simulink library "wt_blockset_beta"  (Simulink 5.0)
values from neighbouring files (symbols this model uses):
  a = -Le\Re    [matrix_coeff_trafo3limb_abc.m]
  a11 = K2*Rs/Ls    [matrix_coeff_scim_abc.m]    (also in matrix_coeff_spsm_dq.m = -Rs*Ksgm_frd/Ksgm_d; matrix_coeff_trafo_abc.m = K2*Rhv/Lhv; matrix_coeff_wrim_abc.m)
  a12 = K3*Rs/Ls    [matrix_coeff_scim_abc.m]    (also in matrix_coeff_spsm_dq.m = Lssq*Ksgm_frd/Ksgm_d; matrix_coeff_trafo_abc.m = K3*Rhv/Lhv; matrix_coeff_wrim_abc.m)
  a13 = 3*Msr*sqrt(3)*K4/4    [matrix_coeff_scim_abc.m]    (also in matrix_coeff_spsm_dq.m = Rf*Lsgm_rd*Lmd/Ksgm_d; matrix_coeff_trafo_abc.m = K4*Rhv; matrix_coeff_wrim_abc.m)
  a14 = K4*Rr    [matrix_coeff_scim_abc.m]    (also in matrix_coeff_spsm_dq.m = Rrd*Lsgm_f*Lmd/Ksgm_d; matrix_coeff_trafo_abc.m = K2/Lhv; matrix_coeff_wrim_abc.m)
  a15 = Msr*(K2-K3)/Ls    [matrix_coeff_scim_abc.m]    (also in matrix_coeff_spsm_dq.m = Lmq*Ksgm_frd/Ksgm_d; matrix_coeff_trafo_abc.m = K3/Lhv; matrix_coeff_wrim_abc.m)
  a16 = K2/Ls    [matrix_coeff_scim_abc.m]    (also in matrix_coeff_spsm_dq.m = Ksgm_frd/Ksgm_d; matrix_coeff_trafo_abc.m = K4; matrix_coeff_wrim_abc.m)
  a17 = K3/Ls    [matrix_coeff_scim_abc.m]    (also in matrix_coeff_spsm_dq.m = -Lsgm_rd*Lmd/Ksgm_d; matrix_coeff_wrim_abc.m)
  a21 = -Lssd*Lsrq/Ksgm_q    [matrix_coeff_spsm_dq.m]
  a22 = -Rs*Lsrq/Ksgm_q    [matrix_coeff_spsm_dq.m]
  a23 = -Lsrq*Lmd/Ksgm_q    [matrix_coeff_spsm_dq.m]
  a24 = -Lsrq*Lmd/Ksgm_q    [matrix_coeff_spsm_dq.m]
  a25 = Rrq*Lmq/Ksgm_q    [matrix_coeff_spsm_dq.m]
  a26 = Lsrq/Ksgm_q    [matrix_coeff_spsm_dq.m]
  a31 = K4*Rs    [matrix_coeff_scim_abc.m]    (also in matrix_coeff_spsm_dq.m = +Rs*Lsgm_rd*Lmd/Ksgm_d; matrix_coeff_trafo_abc.m = K4*Rlv; matrix_coeff_wrim_abc.m)
  a32 = Msr*(K2-K3)/Lr    [matrix_coeff_scim_abc.m]    (also in matrix_coeff_spsm_dq.m = -Lssq*Lsgm_rd*Lmd/Ksgm_d; matrix_coeff_trafo_abc.m = K2*Rlv/Llv; matrix_coeff_wrim_abc.m)
  a33 = K2*Rr/Lr    [matrix_coeff_scim_abc.m]    (also in matrix_coeff_spsm_dq.m = -Rf*Ksgm_srd/Ksgm_d; matrix_coeff_trafo_abc.m = K3*Rlv/Llv; matrix_coeff_wrim_abc.m)
  a34 = K3*Rr/Lr    [matrix_coeff_scim_abc.m]    (also in matrix_coeff_spsm_dq.m = Rrd*Lsgm_s*Lmd/Ksgm_d; matrix_coeff_trafo_abc.m = K4; matrix_coeff_wrim_abc.m)
  a35 = 3*Msr*sqrt(3)*K4/4    [matrix_coeff_scim_abc.m]    (also in matrix_coeff_spsm_dq.m = -Lsgm_rd*Lmd*Lmq/Ksgm_d; matrix_coeff_trafo_abc.m = K2/Llv; matrix_coeff_wrim_abc.m)
  a36 = K4    [matrix_coeff_scim_abc.m]    (also in matrix_coeff_spsm_dq.m = -Lsgm_rd*Lmd/Ksgm_d; matrix_coeff_trafo_abc.m = K3/Llv; matrix_coeff_wrim_abc.m)
  a37 = Ksgm_srd/Ksgm_d    [matrix_coeff_spsm_dq.m]    (also in matrix_coeff_wrim_abc.m = K2/Lr)
  a41 = Rs*Lsgm_f*Lmd/Ksgm_d    [matrix_coeff_spsm_dq.m]
  a42 = -Lsgm_f*Lssq*Lmd/Ksgm_d    [matrix_coeff_spsm_dq.m]
  a43 = Rf*Lsgm_s*Lmd/Ksgm_d    [matrix_coeff_spsm_dq.m]
  a44 = -Rrd*Ksgm_sf/Ksgm_d    [matrix_coeff_spsm_dq.m]
  a45 = -Lsgm_f*Lmd*Lmq/Ksgm_d    [matrix_coeff_spsm_dq.m]
  a46 = -Lsgm_f*Lmd/Ksgm_d    [matrix_coeff_spsm_dq.m]
  a47 = -Lsgm_s*Lmd/Ksgm_d    [matrix_coeff_spsm_dq.m]
  a51 = Lssd*Lmq/Ksgm_q    [matrix_coeff_spsm_dq.m]
  a52 = Rs*Lmq/Ksgm_q    [matrix_coeff_spsm_dq.m]
  a53 = Lmd*Lmq/Ksgm_q    [matrix_coeff_spsm_dq.m]
  a54 = Lmd*Lmq/Ksgm_q    [matrix_coeff_spsm_dq.m]
  a55 = -Rrq*Lssq/Ksgm_q    [matrix_coeff_spsm_dq.m]
  a56 = -Lmq/Ksgm_q    [matrix_coeff_spsm_dq.m]
  alpha_T = Ubase_hv/Ubase_lv    [matrix_coeff_trafo3limb_abc.m]
  b = inv(Le)    [matrix_coeff_trafo3limb_abc.m]
  Ctorque = cq(2:5:102,2:5:182)    [cq_table.m]
  Lmd = mag_ind(1)    [matrix_coeff_spsm_dq.m]
  Lmq = mag_ind(2)    [matrix_coeff_spsm_dq.m]
  Lss = Lsgms+Lm    [init_dbe_dq_scim.m]
  omg_base = 2*pi*rated_fp(1)    [init_dbe_dq_scim.m]    (also in init_dbe_rms_scim.m)
  p = rated_fp(2)    [init_dbe_dq_scim.m]    (also in init_dbe_rms_scim.m)
  Rs = stator(1)    [init_dbe_dq_scim.m]    (also in init_dbe_rms_scim.m; matrix_coeff_scim_abc.m; matrix_coeff_spsm_dq.m = stator_winding(1); matrix_coeff_wrim_abc.m)
  Xs = omg_base*Lss    [init_dbe_dq_scim.m]    (also in init_dbe_rms_scim.m = Xsgm_s+Xm)
undefined symbols (not defined in the file or in its folder): get, j, Kmode, ModeOp, Type, u0
libraries: simulink_extras x12, simulink x4, dspinverses x1, dspmtrx3 x1, dspsigattribs x1, dspspect3 x1
(part 2 of 4)

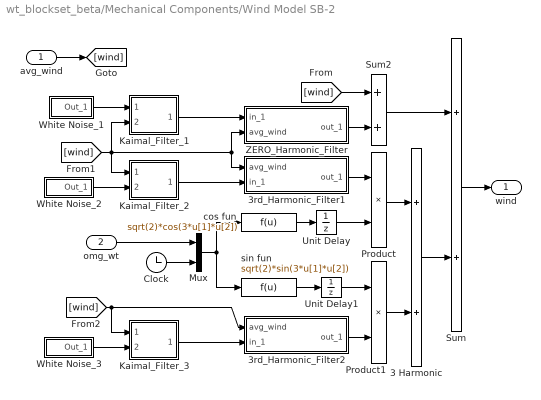
== system wt_blockset_beta/Mechanical Components/Wind Model SB-2 ==
  avg_wind : Inport
  omg_wt : Inport  Port=2
  3 Harmonic : Sum  SaturateOnIntegerOverflow=on  InputSameDT=on
  3rd_Harmonic_Filter1 : Subsystem
  3rd_Harmonic_Filter2 : Subsystem
  Clock : Clock
  Kaimal_Filter_1 : Subsystem
  Kaimal_Filter_2 : Subsystem
  Kaimal_Filter_3 : Subsystem
  Mux : Mux  Inputs=2
  Product : Product  SaturateOnIntegerOverflow=on  InputSameDT=on
  Product1 : Product  SaturateOnIntegerOverflow=on  InputSameDT=on
  Sum : Sum  SaturateOnIntegerOverflow=on  InputSameDT=on
  Sum2 : Sum  SaturateOnIntegerOverflow=on  InputSameDT=on
  Unit Delay : UnitDelay  SampleTime=T_sample
  Unit Delay1 : UnitDelay  SampleTime=T_sample
  White Noise_1 : Subsystem  mask(Continuous White Noise.){Cov=[1], Ts=T_sample, seed=[256]}
      mask prompts: Cov "Noise Power:"; Ts "Sample Time:"
      mask help:
      | White noise for continuous (s-domain) systems.
      | Band-limited using zero-order-hold.
      mask init:
      | r = rand(1,12); r2 = [r(1),r;r,r(12)]; t =[1:13;1:13];
      mask Help: Implemented using white noise into Zero-Order Hold block. The seed and power can be vectors of the same length to produce a vector of white noise sources. For faster simulation, set sample time to the highest value possible but in accordance with the fastest dynamics of system.
      mask Display: plot(t(:),r2(:))
  White Noise_2 : Subsystem  mask(Continuous White Noise.){@1=[1], @2=T_sample, @3=[894]}
      mask prompts: @1 "Noise Power:"; @2 "Sample Time:"; @3 "Seed"
      mask help:
      | White noise for continuous (s-domain) systems.
      | Band-limited using zero-order-hold.
      mask init:
      | Cov = @1; Ts = @2; seed = @3; r = rand(1,12); r2 = [r(1),r;r,r(12)]; t =[1:13;1:13];
      mask Help: Implemented using white noise into Zero-Order Hold block. The seed and power can be vectors of the same length to produce a vector of white noise sources. For faster simulation, set sample time to the highest value possible but in accordance with the fastest dynamics of system.
      mask Display: plot(t(:),r2(:))
  White Noise_3 : Subsystem  mask(Continuous White Noise.){@1=[1], @2=T_sample, @3=[31]}
      mask prompts: @1 "Noise Power:"; @2 "Sample Time:"; @3 "Seed"
      mask help:
      | White noise for continuous (s-domain) systems.
      | Band-limited using zero-order-hold.
      mask init:
      | Cov = @1; Ts = @2; seed = @3; r = rand(1,12); r2 = [r(1),r;r,r(12)]; t =[1:13;1:13];
      mask Help: Implemented using white noise into Zero-Order Hold block. The seed and power can be vectors of the same length to produce a vector of white noise sources. For faster simulation, set sample time to the highest value possible but in accordance with the fastest dynamics of system.
      mask Display: plot(t(:),r2(:))
  ZERO_Harmonic_Filter : Subsystem
  cos fun : Fcn  Expr=sqrt(2)*cos(3*u[1]*u[2])
  sin fun : Fcn  Expr=sqrt(2)*sin(3*u[1]*u[2])
  wind : Outport  InitialOutput=[u0]
  wires:
  Clock/1 -> Mux/2
  Unit Delay1/1 -> Product1/1
  Unit Delay/1 -> Product/2
  omg_wt/1 -> Mux/1
  Mux/1 -> sin fun/1, cos fun/1
  3rd_Harmonic_Filter1/1(out_1) -> Product/1
  White Noise_3/1(Out_1) -> Kaimal_Filter_3/2(in_1)
  White Noise_1/1(Out_1) -> Kaimal_Filter_1/1(in_1)
  Sum/1 -> wind/1
  [wind] -> Sum2/1
  Sum2/1 -> Sum/1
  ZERO_Harmonic_Filter/1(out_1) -> Sum2/2
  3 Harmonic/1 -> Sum/2
  3rd_Harmonic_Filter2/1(out_1) -> Product1/2
  Product1/1 -> 3 Harmonic/2
  Product/1 -> 3 Harmonic/1
  sin fun/1 -> Unit Delay1/1
  cos fun/1 -> Unit Delay/1
  Kaimal_Filter_1/1(out_1) -> ZERO_Harmonic_Filter/1(in_1)
  Kaimal_Filter_2/1(out_1) -> 3rd_Harmonic_Filter1/2(in_1)
  White Noise_2/1(Out_1) -> Kaimal_Filter_2/2(in_1)
  avg_wind/1 -> [wind]
  [wind] -> Kaimal_Filter_1/2(avg_wind), Kaimal_Filter_2/1(avg_wind), ZERO_Harmonic_Filter/2(avg_wind), 3rd_Harmonic_Filter1/1(avg_wind)
  [wind] -> Kaimal_Filter_3/1(avg_wind), 3rd_Harmonic_Filter2/1(avg_wind)
  Kaimal_Filter_3/1(out_1) -> 3rd_Harmonic_Filter2/2(in_1)

== system wt_blockset_beta/Mechanical Components/Wind Turbine Rotor ==
  pitch : Inport
  wind : Inport  Port=2
  omg_wt : Inport  Port=3
  Actuator : TransferFcn  Denominator=[Tact 1]
  Logical Operator : Logic
  Look-Up Table (n-D) : S-Function  FunctionName=sfun_lookupnd  Parameters=numDims,tableData,bp1,bp2,bp3,bp4,bpcell,searchMode,cacheBpFlag,vectorInputFlag,interpMethod,extrapMethod,rangeErrorMode  mask(LookupNDInterp){numDimsPopupSelect=2, bp1=[0:1:20], bp2=[-90:5:90], bp3=[1:3], bp4=[1:3], bpcell={ [1:3], [1:3] }, explicitNumDims=2, searchMode=Binary Search, cacheBpFlag=off, vectorInputFlag=off, tableData=Ctorque, interpMethod=Linear, extrapMethod=None - Clip, rangeErrorMode=Error}
      mask prompts: numDimsPopupSelect "Number of table dimensions:"; bp1 "First input (row) breakpoint set:"; bp2 "Second (column) input breakpoint set:"; bp3 "Third input breakpoint set:"; bp4 "Fourth input breakpoint set:"; bpcell "Fifth..Nth breakpoint sets (cell array):"; explicitNumDims "Explicit number of dimensions:"; searchMode "Index search method:"; cacheBpFlag "Begin index searches using previous index results"; vectorInputFlag "Use one (vector) input port instead of N ports"; tableData "Table data:"; interpMethod "Interpolation method:"; extrapMethod "Extrapolation method:"; rangeErrorMode "Action for out of range input:"
      mask help: Perform n-dimensional interpolated table lookup including index searches. The table is a sampled representation of a function in N variables. Breakpoint sets relate the input values to positions in the table. The first dimension corresponds to the top (or left) input port.
      mask init:
      | if numDimsPopupSelect==5
      |   numDims=explicitNumDims;
      | else
      |   numDims=numDimsPopupSelect;
      | end
      | if strcmp(get_param(bdroot(gcb),'BlockDiagramType'),'library')
      |   dimsChar = 'n';
      | else
      |   dimsChar = sprintf('%d',numDims);
      | end
      | switch interpMethod
      |   case 1
      |     plottype = 'flatplot';
      |   case 2
      |     plottype = 'lineplot';
      |   otherwise
      |     plottype = 'splineplot';
      | end
      | for i=1:numDims
      |   switch( i )
      |     case 1
      |       bp = bp1;
      |     case 2
      |       bp = bp2;
      |     case 3
      |       bp = bp3;
      |     case 4
      |       bp = bp4;
      |     otherwise
      |       bp = bpcell{i-4};
      |    end
      |    Lbp = length(bp);
      |    if i < 2
      |      bpData = reshape(bp,Lbp,1);
      |      bpIndices = 0;
      |    else
      |      bpData = [ bpData; reshape(bp,Lbp,1) ];
      |      bpIndices = [ bpIndices; bpIndices(i-1)+LbpPrev ];
      |    end
      |    LbpPrev = Lbp;
      | end
      | [x,y,xaxes,yaxes] = ndlookico(plottype, numDims,{bpData,bpIndices,tableData});
      mask StyleString: popup(   1   |   2   |   3   |   4   |More...),edit,edit,edit,edit,edit,edit,popup(Evenly Spaced Points|Linear Search|Binary Search),checkbox,checkbox,edit,popup(None - Flat|Linear|Cubic Spline),popup(None - Clip|Linear|Cubic Spline),popup(None|Warning|Error)
      mask CallbackString: ndlookico|||||||||||||
      mask Display:
      | text(0.5,0.9,sprintf(' %s-D T(u)',dimsChar),'horizontalAlignment','center')
      | plot(x,y)
      | plot(xaxes,yaxes)
  Mux : Mux  Inputs=2
  Mux1 : Mux  Inputs=2
  Relational Operator : RelationalOperator  InputSameDT=on
  Relational Operator1 : RelationalOperator  Operator=<=  InputSameDT=on
  Switch : Switch  Threshold=.5  SaturateOnIntegerOverflow=on  InputSameDT=on
  Torque : Fcn  Expr=-0.5*pi*ro_air*(R^3)*(u(1)^2)*u(2)
  cut_in : Constant  Value=cut_in
  cut_out : Constant  Value=cut_out
  lamda : Fcn  Expr=u(2)*R/u(1)
  null : Constant  Value=0
  T_wt : Outport
  wires:
  pitch/1 -> Actuator/1
  lamda/1 -> Look-Up Table (n-D)/1
  Look-Up Table (n-D)/1 -> Mux1/2
  wind/1 -> Mux1/1, Relational Operator1/1, Relational Operator/1, Mux/1
  Logical Operator/1 -> Switch/2
  null/1 -> Switch/3
  Torque/1 -> Switch/1
  Switch/1 -> T_wt/1
  Relational Operator/1 -> Logical Operator/1
  Relational Operator1/1 -> Logical Operator/2
  cut_out/1 -> Relational Operator1/2
  cut_in/1 -> Relational Operator/2
  omg_wt/1 -> Mux/2
  Mux1/1 -> Torque/1
  Mux/1 -> lamda/1
  Actuator/1 -> Look-Up Table (n-D)/2

== system wt_blockset_beta/Power Converters/3-phase Diode Bridge Rectifier ==
  note: Phase Voltage
  note: Phase Current
  note: DC-link Current
  v_ph : Inport
  Idc : Inport  Port=2
  DC-link Voltage : Fcn  Expr=u(1)+u(2)+u(3)
  Diode  State Calculator : Subsystem
  Product1 : Product  SaturateOnIntegerOverflow=on  InputSameDT=on
  Product3 : Product  SaturateOnIntegerOverflow=on  InputSameDT=on
  i_ph : Outport  InitialOutput=0
  Vdc : Outport  Port=2  InitialOutput=0
  wires:
  v_ph/1 -> Diode  State Calculator/1(RST), Product3/1
  Product3/1 -> DC-link Voltage/1
  DC-link Voltage/1 -> Vdc/1
  Diode  State Calculator/1(K) -> Product3/2, Product1/1
  Idc/1 -> Product1/2
  Product1/1 -> i_ph/1

== system wt_blockset_beta/Power Converters/Average PWM Strategy ==
  vd_ref : Inport
  vq_ref : Inport  Port=2
  Vdc : Inport  Port=3
  freq : Inport  Port=4
  Gain : Gain  Gain=2*pi  SaturateOnIntegerOverflow=on
  Integrator : Integrator
  Mux : Mux  Inputs=2
  Mux1 : Mux  Inputs=3
  Mux2 : Mux  Inputs=3
  duty_A1 : Fcn  Expr=0.5*2/sqrt(3)*u(1)*(sin(u(2))+(sin(3*u(2))/6)*(third==1))
  duty_A2 : Fcn  Expr=0.5*2/sqrt(3)*u(1)*(sin(u(2)-2*pi/3)+(sin(3*u(2))/6)*(third==1))
  duty_A3 : Fcn  Expr=0.5*2/sqrt(3)*u(1)*(sin(u(2)+2*pi/3)+(sin(3*u(2))/6)*(third==1))
  ma : Fcn  Expr=sqrt(3)/2*sqrt(u(1)^2+u(3)^2)/u(2)
  duty_ABC : Outport
  wires:
  freq/1 -> Gain/1
  Mux/1 -> duty_A1/1, duty_A2/1, duty_A3/1
  Integrator/1 -> Mux/2
  Gain/1 -> Integrator/1
  duty_A1/1 -> Mux1/1
  duty_A2/1 -> Mux1/2
  duty_A3/1 -> Mux1/3
  Mux2/1 -> ma/1
  ma/1 -> Mux/1
  vd_ref/1 -> Mux2/1  "vdref"
  Vdc/1 -> Mux2/2  "vdc"
  vq_ref/1 -> Mux2/3  "vqref"
  Mux1/1 -> duty_ABC/1

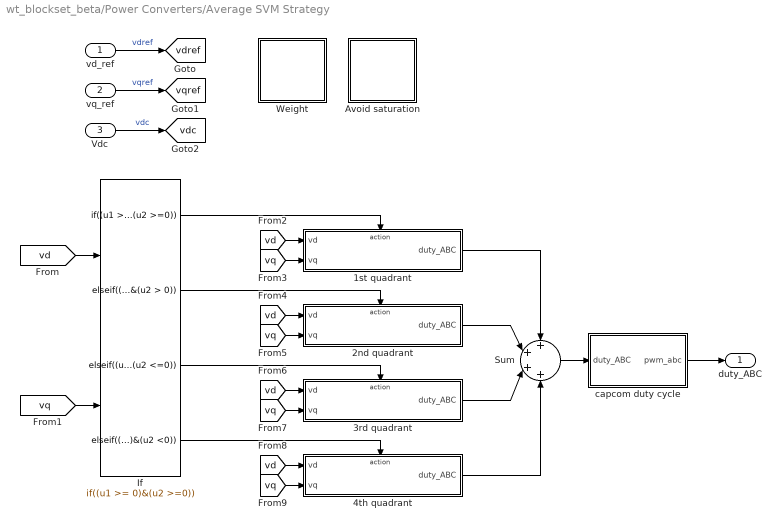
== system wt_blockset_beta/Power Converters/Average SVM Strategy ==
  vd_ref : Inport
  vq_ref : Inport  Port=2
  Vdc : Inport  Port=3
  1st quadrant : Subsystem  TreatAsAtomicUnit=on
  2nd quadrant : Subsystem  TreatAsAtomicUnit=on
  3rd quadrant : Subsystem  TreatAsAtomicUnit=on
  4th quadrant : Subsystem  TreatAsAtomicUnit=on
  "Avoid saturation " : Subsystem
      mask Display: disp('Avoid\nSaturation')
  If : If  NumInputs=2  IfExpression=(u1 >= 0)&(u2 >=0)  ElseIfExpressions=(u1 < 0)&(u2 > 0), (u1 < 0)&(u2 <=0), (u1 >= 0)&(u2 <0)  ShowElse=off
  Sum : Sum  Inputs=++++  SaturateOnIntegerOverflow=on
  Weight : Subsystem
      mask Type: Avoid saturation
      mask Display: disp('Weight')
  capcom duty cycle : Subsystem
  duty_ABC : Outport
  tag scope: vdc=global, vdref=global, vqref=global
  wires:
  vd_ref/1 -> [vdref]  "vdref"
  vq_ref/1 -> [vqref]  "vqref"
  Vdc/1 -> [vdc]  "vdc"
  [vd] -> If/1
  [vq] -> If/2
  If/1 -> 1st quadrant/Action
  [vd] -> 1st quadrant/1(vd)
  [vq] -> 1st quadrant/2(vq)
  [vd] -> 2nd quadrant/1(vd)
  [vq] -> 2nd quadrant/2(vq)
  If/2 -> 2nd quadrant/Action
  [vd] -> 3rd quadrant/1(vd)
  [vq] -> 3rd quadrant/2(vq)
  If/3 -> 3rd quadrant/Action
  [vd] -> 4th quadrant/1(vd)
  [vq] -> 4th quadrant/2(vq)
  If/4 -> 4th quadrant/Action
  1st quadrant/1(duty_ABC) -> Sum/1
  2nd quadrant/1(duty_ABC) -> Sum/2
  4th quadrant/1(duty_ABC) -> Sum/4
  3rd quadrant/1(duty_ABC) -> Sum/3
  Sum/1 -> capcom duty cycle/1(duty_ABC)
  capcom duty cycle/1(pwm_abc) -> duty_ABC/1

== system wt_blockset_beta/Power Converters/Switching PWM Strategy ==
  vd_ref : Inport
  vq_ref : Inport  Port=2
  Vdc : Inport  Port=3
  freq : Inport  Port=4
  Gain : Gain  Gain=2*pi  SaturateOnIntegerOverflow=on
  Integrator : Integrator
  Mux : Mux  Inputs=2
  Mux1 : Mux  Inputs=3
  Mux2 : Mux  Inputs=3
  capcom : Subsystem
  dead_time_A : Subsystem
  duty_A1 : Fcn  Expr=0.5*2/sqrt(3)*u(1)*(sin(u(2))+(sin(3*u(2))/6)*(third==1))
  duty_A2 : Fcn  Expr=0.5*2/sqrt(3)*u(1)*(sin(u(2)-2*pi/3)+(sin(3*u(2))/6)*(third==1))
  duty_A3 : Fcn  Expr=0.5*2/sqrt(3)*u(1)*(sin(u(2)+2*pi/3)+(sin(3*u(2))/6)*(third==1))
  ma : Fcn  Expr=sqrt(3)/2*sqrt(u(1)^2+u(3)^2)/u(2)
  pulse dropping : Subsystem
  Sw_ABC : Outport
  wires:
  vq_ref/1 -> Mux2/3  "vqref"
  Vdc/1 -> Mux2/2  "vdc"
  vd_ref/1 -> Mux2/1  "vdref"
  ma/1 -> Mux/1
  Mux2/1 -> ma/1
  duty_A3/1 -> Mux1/3
  duty_A2/1 -> Mux1/2
  duty_A1/1 -> Mux1/1
  Gain/1 -> Integrator/1
  Integrator/1 -> Mux/2
  Mux/1 -> duty_A3/1, duty_A2/1, duty_A1/1
  freq/1 -> Gain/1
  capcom/1(S_ABC) -> dead_time_A/1(pwm_A)
  Mux1/1 -> pulse dropping/1(duty_ABC)
  pulse dropping/1(duty_abc) -> capcom/1(duty_abc)
  dead_time_A/1(S_A) -> Sw_ABC/1

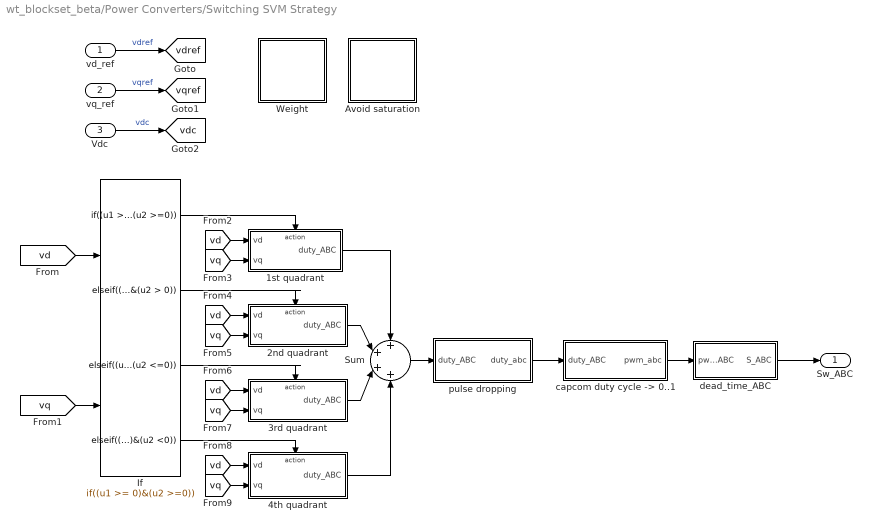
== system wt_blockset_beta/Power Converters/Switching SVM Strategy ==
  vd_ref : Inport
  vq_ref : Inport  Port=2
  Vdc : Inport  Port=3
  1st quadrant : Subsystem  TreatAsAtomicUnit=on
  2nd quadrant : Subsystem  TreatAsAtomicUnit=on
  3rd quadrant : Subsystem  TreatAsAtomicUnit=on
  4th quadrant : Subsystem  TreatAsAtomicUnit=on
  "Avoid saturation " : Subsystem
      mask Display: disp('Avoid\nSaturation')
  If : If  NumInputs=2  IfExpression=(u1 >= 0)&(u2 >=0)  ElseIfExpressions=(u1 < 0)&(u2 > 0), (u1 < 0)&(u2 <=0), (u1 >= 0)&(u2 <0)  ShowElse=off
  Sum : Sum  Inputs=++++  SaturateOnIntegerOverflow=on
  Weight : Subsystem
      mask Type: Avoid saturation
      mask Display: disp('Weight')
  "capcom duty cycle -> 0..1" : Subsystem
  dead_time_ABC : Subsystem
  pulse dropping : Subsystem
  Sw_ABC : Outport
  tag scope: vdc=global, vdref=global, vqref=global
  wires:
  vd_ref/1 -> [vdref]  "vdref"
  vq_ref/1 -> [vqref]  "vqref"
  Vdc/1 -> [vdc]  "vdc"
  [vd] -> If/1
  [vq] -> If/2
  If/1 -> 1st quadrant/Action
  [vd] -> 1st quadrant/1(vd)
  [vq] -> 1st quadrant/2(vq)
  [vd] -> 2nd quadrant/1(vd)
  [vq] -> 2nd quadrant/2(vq)
  If/2 -> 2nd quadrant/Action
  [vd] -> 3rd quadrant/1(vd)
  [vq] -> 3rd quadrant/2(vq)
  If/3 -> 3rd quadrant/Action
  [vd] -> 4th quadrant/1(vd)
  [vq] -> 4th quadrant/2(vq)
  If/4 -> 4th quadrant/Action
  1st quadrant/1(duty_ABC) -> Sum/1
  2nd quadrant/1(duty_ABC) -> Sum/2
  4th quadrant/1(duty_ABC) -> Sum/4
  3rd quadrant/1(duty_ABC) -> Sum/3
  dead_time_ABC/1(S_ABC) -> Sw_ABC/1
  "capcom duty cycle -> 0..1"/1(pwm_abc) -> dead_time_ABC/1(pwm_ABC)
  Sum/1 -> pulse dropping/1(duty_ABC)
  pulse dropping/1(duty_abc) -> "capcom duty cycle -> 0..1"/1(duty_ABC)

== system wt_blockset_beta/Power Converters/Voltage Source Converter ==
  note: DC-link voltage
  note: Commutation functions
  note: Output voltage
  S_ABC : Inport
  Vdc : Inport  Port=2
  i_ph : Inport  Port=3
  DC_link current : Fcn  Expr=u(1)+u(2)+u(3)
  Matrix Gain : Gain  Gain=[2/3 -1/3 -1/3;-1/3 2/3 -1/3;-1/3 -1/3 2/3]  Multiplication=Matrix(u*K)  SaturateOnIntegerOverflow=on
  Product : Product  SaturateOnIntegerOverflow=on  InputSameDT=on
  Product1 : Product  SaturateOnIntegerOverflow=on  InputSameDT=on
  Idc : Outport
  v_ph : Outport  Port=2
  wires:
  Product1/1 -> v_ph/1
  Vdc/1 -> Product1/2
  Matrix Gain/1 -> Product1/1
  S_ABC/1 -> Product/2, Matrix Gain/1
  DC_link current/1 -> Idc/1
  Product/1 -> DC_link current/1
  i_ph/1 -> Product/1

== system wt_blockset_beta/Transformations/ABC->Mag&Phase ==
  ABC : Inport
  Complex to Magnitude-Angle : ComplexToMagnitudeAngle
  Constant : Constant  Value=j*2*pi/3
  Constant1 : Constant  Value=-j*2*pi/3
  Constant3 : Constant  Value=j*0
  Demux : Demux  Outputs=3
  Gain : Gain  Gain=180/pi  SaturateOnIntegerOverflow=on
  Gain1 : Gain  Gain=2/sqrt(2)/3  SaturateOnIntegerOverflow=on
  Gain3 : Gain  Gain=1/3  SaturateOnIntegerOverflow=on
  Math Function : Math
  Math Function1 : Math
  Math Function2 : Math
  Product1 : Product  SaturateOnIntegerOverflow=on  InputSameDT=on
  Product2 : Product  SaturateOnIntegerOverflow=on  InputSameDT=on
  Product4 : Product  SaturateOnIntegerOverflow=on  InputSameDT=on
  Sum : Sum  Inputs=+++  SaturateOnIntegerOverflow=on  InputSameDT=on
  Sum1 : Sum  Inputs=+++  SaturateOnIntegerOverflow=on  InputSameDT=on
  RMS : Outport
  phase : Outport  Port=2
  zero : Outport  Port=3
  wires:
  Constant/1 -> Math Function/1
  Demux/2 -> Product1/1, Sum1/2
  Math Function/1 -> Product1/2
  Constant1/1 -> Math Function1/1
  Demux/3 -> Product2/1, Sum1/3
  Math Function1/1 -> Product2/2
  Product2/1 -> Sum/3
  Product1/1 -> Sum/2
  Complex to Magnitude-Angle/2 -> Gain/1
  Complex to Magnitude-Angle/1 -> Gain1/1
  Gain1/1 -> RMS/1
  ABC/1 -> Demux/1
  Gain/1 -> phase/1
  Product4/1 -> Sum/1
  Demux/1 -> Product4/1, Sum1/1
  Constant3/1 -> Math Function2/1
  Math Function2/1 -> Product4/2
  Sum/1 -> Complex to Magnitude-Angle/1
  Sum1/1 -> Gain3/1
  Gain3/1 -> zero/1

== system wt_blockset_beta/Transformations/DQ -> Complex ==
  A_dq : Inport
  Gain : Gain  Gain=-1  SaturateOnIntegerOverflow=on
  Real-Imag to Complex : RealImagToComplex
  Selector : Selector  Elements=[2]  InputPortWidth=2
  Selector1 : Selector  Elements=[1]  InputPortWidth=2
  A_cmpl : Outport
  wires:
  Real-Imag to Complex/1 -> A_cmpl/1
  A_dq/1 -> Selector/1, Selector1/1
  Selector/1 -> Real-Imag to Complex/1
  Selector1/1 -> Gain/1
  Gain/1 -> Real-Imag to Complex/2

== system wt_blockset_beta/Transformations/abc -> dq0 ==
  ABC : Inport
  theta : Inport  Port=2
  Mux : Mux  Inputs=[3 1]
  Mux1 : Mux  Inputs=3
  v0 : Fcn  Expr=(u(1)+u(2)+u(3))/3
  vd : Fcn  Expr=2*(u[1]*cos(u[4])+u[2]*cos(u[4]-2*pi/3)+u[3]*cos(u[4]+2*pi/3))/3
  vq : Fcn  Expr=-2*(u[1]*sin(u[4])+u[2]*sin(u[4]-2*pi/3)+u[3]*sin(u[4]+2*pi/3))/3
  DQO : Outport  InitialOutput=0
  wires:
  theta/1 -> Mux/2
  Mux1/1 -> DQO/1
  Mux/1 -> vd/1, vq/1, v0/1
  ABC/1 -> Mux/1
  vd/1 -> Mux1/1
  vq/1 -> Mux1/2
  v0/1 -> Mux1/3

== system wt_blockset_beta/Transformations/dq0 -> abc ==
  DQO : Inport
  theta : Inport  Port=2
  Mux : Mux  Inputs=[3 1]
  Mux1 : Mux  Inputs=3
  va : Fcn  Expr=u[1]*cos(u[4])-u[2]*sin(u[4])+u(3)
  vb : Fcn  Expr=u[1]*cos(u[4]-2*pi/3)-u[2]*sin(u[4]-2*pi/3)+u(3)
  vc : Fcn  Expr=u[1]*cos(u[4]+2*pi/3)-u[2]*sin(u[4]+2*pi/3)+u(3)
  ABC : Outport  InitialOutput=0
  wires:
  theta/1 -> Mux/2
  Mux1/1 -> ABC/1
  vc/1 -> Mux1/3
  vb/1 -> Mux1/2
  va/1 -> Mux1/1
  DQO/1 -> Mux/1
  Mux/1 -> va/1, vb/1, vc/1

== system wt_blockset_beta/Transformations/phase -> line currents ==
  i_phase : Inport
  phase ->line currents : Gain  Gain=[1 0 -1;-1 1 0;0 -1 1]  Multiplication=Matrix(K*u)  SaturateOnIntegerOverflow=on
  i_line : Outport
  wires:
  i_phase/1 -> phase ->line currents/1
  phase ->line currents/1 -> i_line/1

== system wt_blockset_beta/Transformations/phase->line voltages ==
  v_phase : Inport
  phase ->line voltages : Gain  Gain=[1 -1 0; 0 1 -1; -1 0 1]  Multiplication=Matrix(K*u)  SaturateOnIntegerOverflow=on
  v_line : Outport
  wires:
  phase ->line voltages/1 -> v_line/1
  v_phase/1 -> phase ->line voltages/1

== system wt_blockset_beta/Common Models/3-phase 3 limb  C S-Function/phase->line2 ==
  in : Inport
  Mux1 : Mux  Inputs=3
  ab : Fcn  Expr=u(1)-u(3)
  bc : Fcn  Expr=u(2)-u(1)
  ca : Fcn  Expr=u(3)-u(2)
  out : Outport
  wires:
  in/1 -> bc/1, ca/1, ab/1
  Mux1/1 -> out/1
  ca/1 -> Mux1/3
  bc/1 -> Mux1/2
  ab/1 -> Mux1/1

== system wt_blockset_beta/Common Models/3-phase 3 limb  Transformer/phase->line2 ==
  in : Inport
  Mux1 : Mux  Inputs=3
  ab : Fcn  Expr=u(1)-u(3)
  bc : Fcn  Expr=u(2)-u(1)
  ca : Fcn  Expr=u(3)-u(2)
  out : Outport
  wires:
  ab/1 -> Mux1/1
  bc/1 -> Mux1/2
  ca/1 -> Mux1/3
  Mux1/1 -> out/1
  in/1 -> ab/1, ca/1, bc/1

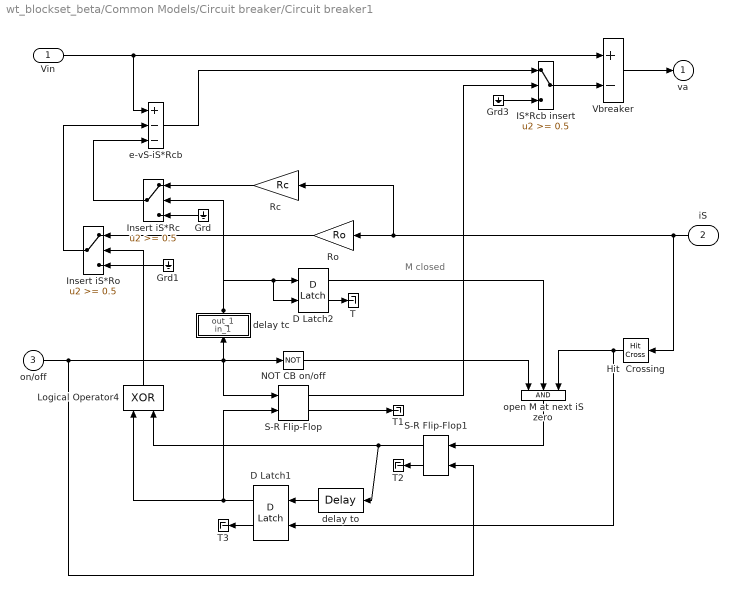
== system wt_blockset_beta/Common Models/Circuit breaker/Circuit breaker1 ==
  note: M closed
  Vin : Inport
  iS : Inport  Orientation=left  Port=2
  on/off : Inport  Port=3
  D Latch1 : simulink_extras/Flip Flops/D Latch  Orientation=left
  D Latch2 : simulink_extras/Flip Flops/D Latch
  Grd : Ground  Orientation=left
  Grd1 : Ground  Orientation=left
  Grd3 : Ground
  Hit  Crossing : HitCross  Orientation=left
  IS*Rcb insert : Switch  Threshold=0.5  SaturateOnIntegerOverflow=on  InputSameDT=on
  Insert iS*Rc : Switch  Orientation=left  Threshold=0.5  SaturateOnIntegerOverflow=on  InputSameDT=on
  Insert iS*Ro : Switch  Orientation=left  Threshold=0.5  SaturateOnIntegerOverflow=on  InputSameDT=on
  Logical Operator4 : Logic  Orientation=up  Operator=XOR
  NOT CB on/off : Logic  Operator=NOT  Inputs=1
  Rc : Gain  Orientation=left  Gain=Rc  SaturateOnIntegerOverflow=on
  Ro : Gain  Orientation=left  Gain=Ro  SaturateOnIntegerOverflow=on
  S-R Flip-Flop : simulink_extras/Flip Flops/S-R Flip-Flop  initial_condition=0
  S-R Flip-Flop1 : simulink_extras/Flip Flops/S-R Flip-Flop  Orientation=left  initial_condition=0
  T{,1..3} (4 alike) : Terminator
  Vbreaker : Sum  Inputs=+-  SaturateOnIntegerOverflow=on  InputSameDT=on
  delay tc : Subsystem  Orientation=up
  delay to : TransportDelay  Orientation=left  DelayTime=to  BufferSize=20000
  e-vS-iS*Rcb : Sum  Inputs=+--  SaturateOnIntegerOverflow=on  InputSameDT=on
  open M at next iS zero : Logic  Orientation=down  Inputs=3
  va : Outport
  wires:
  Ro/1 -> Insert iS*Ro/1
  e-vS-iS*Rcb/1 -> IS*Rcb insert/1
  Rc/1 -> Insert iS*Rc/1
  Insert iS*Ro/1 -> e-vS-iS*Rcb/2
  Insert iS*Rc/1 -> e-vS-iS*Rcb/3
  on/off/1 -> NOT CB on/off/1, S-R Flip-Flop1/2, delay tc/1(in_1), S-R Flip-Flop/1
  delay tc/1(out_1) -> D Latch2/1, D Latch2/2, Insert iS*Rc/2
  Logical Operator4/1 -> Insert iS*Ro/2
  Grd/1 -> Insert iS*Rc/3
  Grd1/1 -> Insert iS*Ro/3
  D Latch2/2 -> T/1
  delay to/1 -> D Latch1/1
  S-R Flip-Flop1/1 -> Logical Operator4/2, delay to/1
  S-R Flip-Flop1/2 -> T2/1
  Hit  Crossing/1 -> open M at next iS zero/3, D Latch1/2
  D Latch1/2 -> T3/1
  D Latch1/1 -> Logical Operator4/1, S-R Flip-Flop/2
  D Latch2/1 -> open M at next iS zero/2
  NOT CB on/off/1 -> open M at next iS zero/1
  open M at next iS zero/1 -> S-R Flip-Flop1/1
  Vbreaker/1 -> va/1
  IS*Rcb insert/1 -> Vbreaker/2
  Grd3/1 -> IS*Rcb insert/3
  Vin/1 -> Vbreaker/1, e-vS-iS*Rcb/1
  iS/1 -> Ro/1, Rc/1, Hit  Crossing/1
  S-R Flip-Flop/2 -> T1/1
  S-R Flip-Flop/1 -> IS*Rcb insert/2

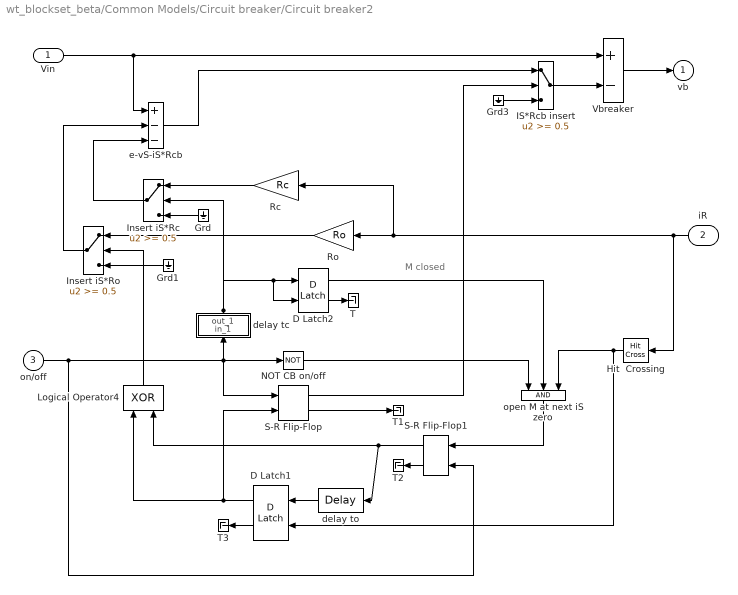
== system wt_blockset_beta/Common Models/Circuit breaker/Circuit breaker2 ==
  note: M closed
  Vin : Inport
  iR : Inport  Orientation=left  Port=2
  on/off : Inport  Port=3
  D Latch1 : simulink_extras/Flip Flops/D Latch  Orientation=left
  D Latch2 : simulink_extras/Flip Flops/D Latch
  Grd : Ground  Orientation=left
  Grd1 : Ground  Orientation=left
  Grd3 : Ground
  Hit  Crossing : HitCross  Orientation=left
  IS*Rcb insert : Switch  Threshold=0.5  SaturateOnIntegerOverflow=on  InputSameDT=on
  Insert iS*Rc : Switch  Orientation=left  Threshold=0.5  SaturateOnIntegerOverflow=on  InputSameDT=on
  Insert iS*Ro : Switch  Orientation=left  Threshold=0.5  SaturateOnIntegerOverflow=on  InputSameDT=on
  Logical Operator4 : Logic  Orientation=up  Operator=XOR
  NOT CB on/off : Logic  Operator=NOT  Inputs=1
  Rc : Gain  Orientation=left  Gain=Rc  SaturateOnIntegerOverflow=on
  Ro : Gain  Orientation=left  Gain=Ro  SaturateOnIntegerOverflow=on
  S-R Flip-Flop : simulink_extras/Flip Flops/S-R Flip-Flop  initial_condition=0
  S-R Flip-Flop1 : simulink_extras/Flip Flops/S-R Flip-Flop  Orientation=left  initial_condition=0
  T{,1..3} (4 alike) : Terminator
  Vbreaker : Sum  Inputs=+-  SaturateOnIntegerOverflow=on  InputSameDT=on
  delay tc : Subsystem  Orientation=up
  delay to : TransportDelay  Orientation=left  DelayTime=to  BufferSize=20000
  e-vS-iS*Rcb : Sum  Inputs=+--  SaturateOnIntegerOverflow=on  InputSameDT=on
  open M at next iS zero : Logic  Orientation=down  Inputs=3
  vb : Outport
  wires:
  S-R Flip-Flop/1 -> IS*Rcb insert/2
  S-R Flip-Flop/2 -> T1/1
  iR/1 -> Hit  Crossing/1, Rc/1, Ro/1
  Vin/1 -> e-vS-iS*Rcb/1, Vbreaker/1
  Grd3/1 -> IS*Rcb insert/3
  IS*Rcb insert/1 -> Vbreaker/2
  Vbreaker/1 -> vb/1
  open M at next iS zero/1 -> S-R Flip-Flop1/1
  NOT CB on/off/1 -> open M at next iS zero/1
  D Latch2/1 -> open M at next iS zero/2
  D Latch1/1 -> S-R Flip-Flop/2, Logical Operator4/1
  D Latch1/2 -> T3/1
  Hit  Crossing/1 -> D Latch1/2, open M at next iS zero/3
  S-R Flip-Flop1/2 -> T2/1
  S-R Flip-Flop1/1 -> delay to/1, Logical Operator4/2
  delay to/1 -> D Latch1/1
  D Latch2/2 -> T/1
  Grd1/1 -> Insert iS*Ro/3
  Grd/1 -> Insert iS*Rc/3
  Logical Operator4/1 -> Insert iS*Ro/2
  delay tc/1(out_1) -> Insert iS*Rc/2, D Latch2/2, D Latch2/1
  on/off/1 -> S-R Flip-Flop/1, delay tc/1(in_1), S-R Flip-Flop1/2, NOT CB on/off/1
  Insert iS*Rc/1 -> e-vS-iS*Rcb/3
  Insert iS*Ro/1 -> e-vS-iS*Rcb/2
  Rc/1 -> Insert iS*Rc/1
  e-vS-iS*Rcb/1 -> IS*Rcb insert/1
  Ro/1 -> Insert iS*Ro/1

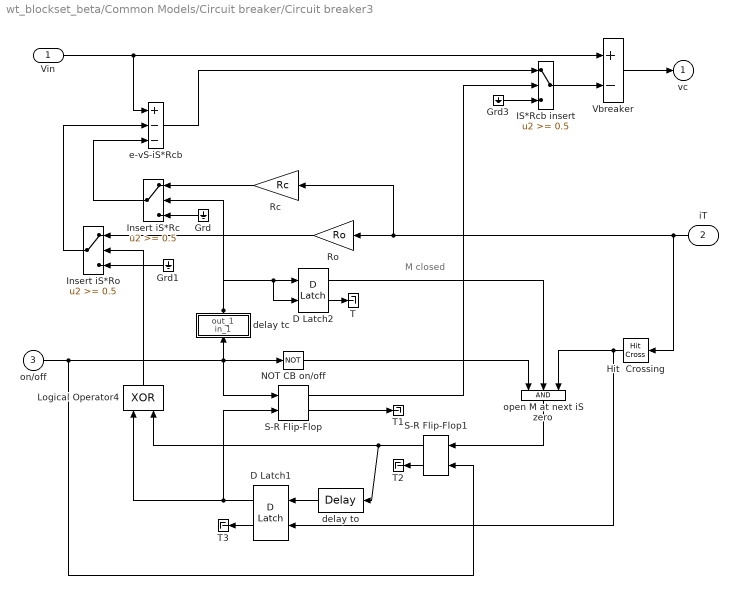
== system wt_blockset_beta/Common Models/Circuit breaker/Circuit breaker3 ==
  note: M closed
  Vin : Inport
  iT : Inport  Orientation=left  Port=2
  on/off : Inport  Port=3
  D Latch1 : simulink_extras/Flip Flops/D Latch  Orientation=left
  D Latch2 : simulink_extras/Flip Flops/D Latch
  Grd : Ground  Orientation=left
  Grd1 : Ground  Orientation=left
  Grd3 : Ground
  Hit  Crossing : HitCross  Orientation=left
  IS*Rcb insert : Switch  Threshold=0.5  SaturateOnIntegerOverflow=on  InputSameDT=on
  Insert iS*Rc : Switch  Orientation=left  Threshold=0.5  SaturateOnIntegerOverflow=on  InputSameDT=on
  Insert iS*Ro : Switch  Orientation=left  Threshold=0.5  SaturateOnIntegerOverflow=on  InputSameDT=on
  Logical Operator4 : Logic  Orientation=up  Operator=XOR
  NOT CB on/off : Logic  Operator=NOT  Inputs=1
  Rc : Gain  Orientation=left  Gain=Rc  SaturateOnIntegerOverflow=on
  Ro : Gain  Orientation=left  Gain=Ro  SaturateOnIntegerOverflow=on
  S-R Flip-Flop : simulink_extras/Flip Flops/S-R Flip-Flop  initial_condition=0
  S-R Flip-Flop1 : simulink_extras/Flip Flops/S-R Flip-Flop  Orientation=left  initial_condition=0
  T{,1..3} (4 alike) : Terminator
  Vbreaker : Sum  Inputs=+-  SaturateOnIntegerOverflow=on  InputSameDT=on
  delay tc : Subsystem  Orientation=up
  delay to : TransportDelay  Orientation=left  DelayTime=to  BufferSize=20000
  e-vS-iS*Rcb : Sum  Inputs=+--  SaturateOnIntegerOverflow=on  InputSameDT=on
  open M at next iS zero : Logic  Orientation=down  Inputs=3
  vc : Outport
  wires:
  Ro/1 -> Insert iS*Ro/1
  e-vS-iS*Rcb/1 -> IS*Rcb insert/1
  Rc/1 -> Insert iS*Rc/1
  Insert iS*Ro/1 -> e-vS-iS*Rcb/2
  Insert iS*Rc/1 -> e-vS-iS*Rcb/3
  on/off/1 -> NOT CB on/off/1, S-R Flip-Flop1/2, delay tc/1(in_1), S-R Flip-Flop/1
  delay tc/1(out_1) -> D Latch2/1, D Latch2/2, Insert iS*Rc/2
  Logical Operator4/1 -> Insert iS*Ro/2
  Grd/1 -> Insert iS*Rc/3
  Grd1/1 -> Insert iS*Ro/3
  D Latch2/2 -> T/1
  delay to/1 -> D Latch1/1
  S-R Flip-Flop1/1 -> Logical Operator4/2, delay to/1
  S-R Flip-Flop1/2 -> T2/1
  Hit  Crossing/1 -> open M at next iS zero/3, D Latch1/2
  D Latch1/2 -> T3/1
  D Latch1/1 -> Logical Operator4/1, S-R Flip-Flop/2
  D Latch2/1 -> open M at next iS zero/2
  NOT CB on/off/1 -> open M at next iS zero/1
  open M at next iS zero/1 -> S-R Flip-Flop1/1
  Vbreaker/1 -> vc/1
  IS*Rcb insert/1 -> Vbreaker/2
  Grd3/1 -> IS*Rcb insert/3
  Vin/1 -> Vbreaker/1, e-vS-iS*Rcb/1
  iT/1 -> Ro/1, Rc/1, Hit  Crossing/1
  S-R Flip-Flop/2 -> T1/1
  S-R Flip-Flop/1 -> IS*Rcb insert/2

== system wt_blockset_beta/Common Models/Harmonic Voltage Source/Phase A ==
  Input : Inport
  Constant1 : Constant  Value=[gama_0;0;0;0;0;0;0]
  Constant2 : Constant  Value=0
  Demux : Demux  Outputs=2
  Product : Product  SaturateOnIntegerOverflow=on
  Selector : Selector  Elements=[1]  InputPortWidth=7
  Sum1 : Sum  Inputs=|++  SaturateOnIntegerOverflow=on
  Sum3 : Sum  Inputs=|++  SaturateOnIntegerOverflow=on
  Sum4 : Sum  Inputs=1  SaturateOnIntegerOverflow=on
  Trigonometric Function : Trigonometry
  amplitudes : Gain  Gain=sqrt(2)*[1;0.05; 0.06; 0.05;0.015;0.035;0.03]  SaturateOnIntegerOverflow=on
  enable : Gain  Gain=[1; h3;h5;h7;h9;h11;h13]  SaturateOnIntegerOverflow=on
  order : Gain  Gain=[1;3;5;7;9;11;13]  SaturateOnIntegerOverflow=on
  v_harm : Outport
  tag scope: gama=global
  wires:
  Sum3/1 -> order/1
  Product/1 -> enable/1
  Sum4/1 -> v_harm/1
  Constant2/1 -> Sum3/2
  Trigonometric Function/1 -> Product/2
  amplitudes/1 -> Product/1
  order/1 -> Sum1/1
  Constant1/1 -> Sum1/2
  Input/1 -> Demux/1
  Demux/1 -> amplitudes/1
  Demux/2 -> Sum3/1
  enable/1 -> Sum4/1
  Selector/1 -> [gama]
  Sum1/1 -> Trigonometric Function/1, Selector/1

== system wt_blockset_beta/Common Models/Harmonic Voltage Source/Phase B ==
  Input : Inport
  Constant1 : Constant  Value=[gama_0;0;0;0;0;0;0]
  Constant2 : Constant  Value=-2*pi/3
  Demux : Demux  Outputs=2
  Product : Product  SaturateOnIntegerOverflow=on
  Sum1 : Sum  Inputs=|++  SaturateOnIntegerOverflow=on
  Sum3 : Sum  Inputs=|++  SaturateOnIntegerOverflow=on
  Sum4 : Sum  Inputs=1  SaturateOnIntegerOverflow=on
  Trigonometric Function : Trigonometry
  amplitudes : Gain  Gain=sqrt(2)*[1;0.05; 0.06; 0.05;0.015;0.035;0.03]  SaturateOnIntegerOverflow=on
  enable : Gain  Gain=[1; h3;h5;h7;h9;h11;h13]  SaturateOnIntegerOverflow=on
  order : Gain  Gain=[1;3;5;7;9;11;13]  SaturateOnIntegerOverflow=on
  v_harm : Outport
  wires:
  Demux/2 -> Sum3/1
  Demux/1 -> amplitudes/1
  Input/1 -> Demux/1
  Constant1/1 -> Sum1/2
  Sum1/1 -> Trigonometric Function/1
  order/1 -> Sum1/1
  amplitudes/1 -> Product/1
  Trigonometric Function/1 -> Product/2
  Constant2/1 -> Sum3/2
  Sum4/1 -> v_harm/1
  Product/1 -> enable/1
  Sum3/1 -> order/1
  enable/1 -> Sum4/1

== system wt_blockset_beta/Common Models/Harmonic Voltage Source/Phase C ==
  Input : Inport
  Constant1 : Constant  Value=[gama_0;0;0;0;0;0;0]
  Constant2 : Constant  Value=+2*pi/3
  Demux : Demux  Outputs=2
  Product : Product  SaturateOnIntegerOverflow=on
  Sum1 : Sum  Inputs=|++  SaturateOnIntegerOverflow=on
  Sum3 : Sum  Inputs=|++  SaturateOnIntegerOverflow=on
  Sum4 : Sum  Inputs=1  SaturateOnIntegerOverflow=on
  Trigonometric Function : Trigonometry
  amplitudes : Gain  Gain=sqrt(2)*[1;0.05; 0.06; 0.05;0.015;0.035;0.03]  SaturateOnIntegerOverflow=on
  enable : Gain  Gain=[1; h3;h5;h7;h9;h11;h13]  SaturateOnIntegerOverflow=on
  order : Gain  Gain=[1;3;5;7;9;11;13]  SaturateOnIntegerOverflow=on
  v_harm : Outport
  wires:
  Sum3/1 -> order/1
  Product/1 -> enable/1
  Sum4/1 -> v_harm/1
  Constant2/1 -> Sum3/2
  Trigonometric Function/1 -> Product/2
  amplitudes/1 -> Product/1
  order/1 -> Sum1/1
  Sum1/1 -> Trigonometric Function/1
  Constant1/1 -> Sum1/2
  Input/1 -> Demux/1
  Demux/1 -> amplitudes/1
  Demux/2 -> Sum3/1
  enable/1 -> Sum4/1

== system wt_blockset_beta/Electrical Machinery/Simulink Blocks  based Models/RMS Wound Rotor Induction Machine ==
  note: Comple steady state model for induction machine.
      | Deep-bar effect is taken into account
  Vs_c : Inport
  Vr_c : Inport  Port=2
  omg_mec : Inport  Port=3
  " LU Inverse" : dspinverses/ LU Inverse
  Complex to Real-Imag : ComplexToRealImag  Output=Real
  Gain : Gain  Gain=3*p*Xm/omg_synch/2  SaturateOnIntegerOverflow=on
  Gain3 : Gain  Gain=p  SaturateOnIntegerOverflow=on
  Impedance Matrix : Subsystem
  Math Function : Math  Operator=conj
  Matrix Concatenation : S-Function  FunctionName=smatrxcat  Parameters=numInports,catMethod  mask(Matrix Concatenation){numInports=2, catMethod=Vertical}
      mask prompts: numInports "Number of inputs:"; catMethod "Concatenation method:"
      mask help: Perform horizontal or vertical concatenation. 1-D vector input signals are treated as column vectors, i.e., [Mx1] matrices. The output is always a matrix.
      mask init:
      | xy = matrxcatmask('icon');
      mask StyleString: edit,popup(Horizontal|Vertical)
      mask Display:
      | plot(xy.x,xy.y);
      | text(0.15,0.86,xy.label);
  Matrix Multiply : dspmtrx3/Matrix Multiply  numInputPorts=2  OptimizationLevel=None
  Product : Product  Inputs=3  SaturateOnIntegerOverflow=on  InputSameDT=on
  Selector Ir : Selector  Elements=[2]  InputPortWidth=2
  Selector Is : Selector  Elements=[1]  InputPortWidth=2
  op : Constant  Value=j
  Is_c : Outport
  Ir_c : Outport  Port=2
  Te : Outport  Port=3
  wires:
  Gain3/1 -> Impedance Matrix/1(omg)
  Gain/1 -> Te/1
  Complex to Real-Imag/1 -> Gain/1
  op/1 -> Product/3
  Product/1 -> Complex to Real-Imag/1
  Selector Ir/1 -> Ir_c/1, Product/2
  Math Function/1 -> Product/1
  Selector Is/1 -> Is_c/1, Math Function/1
  Matrix Multiply/1 -> Selector Ir/1, Selector Is/1
  Matrix Concatenation/1 -> Matrix Multiply/2
  " LU Inverse"/1 -> Matrix Multiply/1
  Impedance Matrix/1(Z) -> " LU Inverse"/1
  omg_mec/1 -> Gain3/1  "slip"
  Vr_c/1 -> Matrix Concatenation/2
  Vs_c/1 -> Matrix Concatenation/1

== system wt_blockset_beta/Electrical Machinery/Simulink Blocks  based Models/RMS  Squirrel Cage Induction Machine ==
  Vs : Inport
  omg_mec : Inport  Port=2
  Gain3 : Gain  Gain=p  SaturateOnIntegerOverflow=on
  Steady State Model : Subsystem
  Is : Outport  InitialOutput=0
  Te : Outport  Port=2  InitialOutput=0
  wires:
  Steady State Model/2(Iph) -> Is/1
  Steady State Model/1(Te) -> Te/1
  Gain3/1 -> Steady State Model/2(omg)
  Vs/1 -> Steady State Model/1(Vs)
  omg_mec/1 -> Gain3/1

== system wt_blockset_beta/Electrical Machinery/Simulink Blocks  based Models/Reduced Order Model Induction Machine ==
  vdq_s : Inport
  vdq_r : Inport  Port=2
  omg_mec : Inport  Port=3
  Gain : Gain  Gain=Q  Multiplication=Matrix(K*u)  SaturateOnIntegerOverflow=on
  Mux : Mux  Inputs=[1 1 2 2 1]
  Mux1 : Mux  Inputs=[1 1 2]
  OpType : Gain  Gain=-1  SaturateOnIntegerOverflow=on
  Reshape : S-Function  FunctionName=sreshape  Parameters=OutputDimensionality, OutputDimensions  mask(Reshape){OutputDimensionality=Column vector, OutputDimensions=[1,1]}
      mask prompts: OutputDimensionality "Output dimensionality:"; OutputDimensions "Output dimensions:"
      mask help:
      | Change the dimensions of a vector or matrix input signal. Output
      |  - a one-dimensional array (vector),
      |  - a column vector (Mx1 matrix),
      |  - a row vector (1xN matrix), or
      |  - a matrix or vector with specified dimensions, e.g., [M, N] or [W].
      mask init:
      | s = reshapemask(gcb,'init');
      mask StyleString: popup(1-D array|Column vector|Row vector|Customize),edit
      mask CallbackString: reshapemask(gcb,'cbDimensionality')|
      mask Display: plot(s.x1,s.y1,s.xc,s.yc);
  Selector : Selector  Elements=[1 2]  InputPortWidth=7
  Te_dyn : Fcn  Expr=1.5*p*Lm*(u(2)*u(3)-u(1)*u(4))/D
  dfi_dr : Integrator  InitialCondition=init_cond(1)
  dfi_qr : Integrator  InitialCondition=init_cond(2)
  fi_dr : Fcn  Expr=tau_rm*(alpha*sigma_r-1/sigma_s)*u(1)+(alpha*omg_e*tau_rm*Lm/tau_sr+omg_e-u(7))*u(2)+alpha*omg_e*tau_rm*u(4)/(tau_sr^2)+alpha*tau_rm*u(3)/tau_sr+u(5)
  fi_ds : Fcn  Expr=alpha*(sigma_r*u(1)+omg_e*Lm/tau_sr*u(2)+omg_e*u(4)/(tau_sr^2)+u(3)/tau_sr)
  fi_qr : Fcn  Expr=-(alpha*omg_e*tau_rm*Lm/tau_sr+omg_e-u(7))*u(1)+tau_rm*(alpha*sigma_r-1/sigma_s)*u(2)+alpha*tau_rm*u(4)/tau_sr-alpha*omg_e*tau_rm*u(3)/(tau_sr^2)+u(6)
  fi_qs : Fcn  Expr=alpha*(-omg_e*Lm*u(1)/tau_sr+sigma_r*u(2)+u(4)/tau_sr-omg_e*u(3)/(tau_sr^2))
  p : Gain  Gain=p  SaturateOnIntegerOverflow=on
  sel_1 : Selector  Elements=[1 2]  InputPortWidth=4
  sel_2 : Selector  Elements=[3 4]  InputPortWidth=4
  idq_s : Outport
  idq_r : Outport  Port=2
  Te : Outport  Port=3
  wires:
  dfi_dr/1 -> Mux/1
  dfi_qr/1 -> Mux/2
  Mux/1 -> fi_dr/1, fi_qr/1, fi_ds/1, fi_qs/1, Selector/1
  fi_dr/1 -> dfi_dr/1
  fi_qr/1 -> dfi_qr/1
  fi_ds/1 -> Mux1/1
  fi_qs/1 -> Mux1/2
  Selector/1 -> Mux1/3
  Mux1/1 -> Te_dyn/1, Reshape/1
  Reshape/1 -> Gain/1
  p/1 -> Mux/5
  omg_mec/1 -> p/1
  vdq_s/1 -> OpType/1
  vdq_r/1 -> Mux/4
  Te_dyn/1 -> Te/1
  sel_1/1 -> idq_s/1
  Gain/1 -> sel_1/1, sel_2/1
  sel_2/1 -> idq_r/1
  OpType/1 -> Mux/3

== system wt_blockset_beta/Electrical Machinery/Simulink Blocks  based Models/Salient-Pole Synchronous Machine constant parameters ==
  note: Generalized model of synchronous machine in rotor reference frame
  vs_UVW : Inport
  vf : Inport  Port=2
  omg_mec : Inport  Port=3
  Gain2 : Gain  Gain=p  SaturateOnIntegerOverflow=on
  Integrator1 : Integrator
  Mathematical model : Subsystem
  abc-dq : Subsystem
  Te : Outport  InitialOutput=0
  is_UVW : Outport  Port=2  InitialOutput=0
  tag scope: theta=global
  wires:
  vs_UVW/1 -> abc-dq/1(ABC)
  Integrator1/1 -> [theta]
  [theta] -> abc-dq/2(theta)
  abc-dq/1(DQ) -> Mathematical model/1(usdq)
  vf/1 -> Mathematical model/2(uf)
  Mathematical model/1(Te) -> Te/1
  omg_mec/1 -> Gain2/1
  Gain2/1 -> Mathematical model/3(omgr), Integrator1/1
  Mathematical model/2(is_UVW) -> is_UVW/1

== system wt_blockset_beta/Electrical Machinery/Simulink Blocks  based Models/Squirrel Cage Induction Machine constant parameters ==
  vs_UVW : Inport
  omg_mec : Inport  Port=2
  Connection Type : Constant  Value=Type
  Derivatives : Subsystem
  Gain3 : Gain  Gain=p  SaturateOnIntegerOverflow=on
  Switch : Switch  SaturateOnIntegerOverflow=on  InputSameDT=on
  abc-dq : Subsystem
  dq / abc : Subsystem
  mode : Gain  Gain=Kmode  SaturateOnIntegerOverflow=on
  phase ->line : Subsystem
  is_UVW : Outport  InitialOutput=0
  Te : Outport  Port=2  InitialOutput=0
  wires:
  [theta] -> dq / abc/2(theta)
  Derivatives/1(idqs) -> dq / abc/1(DQ)
  Derivatives/2(Te) -> Te/1
  Gain3/1 -> Derivatives/2(omega)
  abc-dq/1(DQ) -> Derivatives/1(vdqs)
  vs_UVW/1 -> mode/1
  omg_mec/1 -> Gain3/1
  [theta] -> abc-dq/2(theta)
  mode/1 -> abc-dq/1(ABC)
  phase ->line/1(Out) -> Switch/3
  Connection Type/1 -> Switch/2
  Switch/1 -> is_UVW/1
  dq / abc/1(ABC) -> Switch/1, phase ->line/1(In)

== system wt_blockset_beta/Electrical Machinery/Simulink Blocks  based Models/Squirrel Cage  Induction Machine  with Deep Bar Effect ==
  vs_UVW : Inport
  omg_mec : Inport  Port=2
  Connection Type : Constant  Value=Type
  Derivatives : Subsystem
  Gain3 : Gain  Gain=p  SaturateOnIntegerOverflow=on
  Subsystem1 : Subsystem
  Switch : Switch  SaturateOnIntegerOverflow=on  InputSameDT=on
  abc-dq : Subsystem
  mode : Gain  Gain=Kmode  SaturateOnIntegerOverflow=on
  phase ->line : Subsystem
  is_UVW : Outport  InitialOutput=0
  Te : Outport  Port=2  InitialOutput=0
  wires:
  [theta] -> Subsystem1/2(theta)
  Derivatives/1(idqs) -> Subsystem1/1(DQ)
  Derivatives/2(Te) -> Te/1
  Gain3/1 -> Derivatives/2(omega)
  abc-dq/1(DQ) -> Derivatives/1(vdqs)
  vs_UVW/1 -> mode/1
  omg_mec/1 -> Gain3/1
  [theta] -> abc-dq/2(theta)
  mode/1 -> abc-dq/1(ABC)
  phase ->line/1(Out) -> Switch/3
  Connection Type/1 -> Switch/2
  Switch/1 -> is_UVW/1
  Subsystem1/1(ABC) -> phase ->line/1(In), Switch/1

== system wt_blockset_beta/Electrical Machinery/Simulink Blocks  based Models/Wound Rotor Induction Machine constant parameters ==
  vs_UVW : Inport
  vr_KLM : Inport  Port=2
  omg_mec : Inport  Port=3
  Constant : Constant  Value=0
  Constant1 : Constant  Value=0
  Gain1 : Gain  Gain=p  SaturateOnIntegerOverflow=on
  Subsystem1 : Subsystem
  Subsystem2 : Subsystem
  Voltage equations : Subsystem
  abc-dq : Subsystem
  abc-dq1 : Subsystem
  is_UVW : Outport  InitialOutput=0
  ir_KLM : Outport  Port=2  InitialOutput=0
  Te : Outport  Port=3  InitialOutput=0
  wires:
  Voltage equations/3(Te) -> Te/1
  Voltage equations/2(idqr) -> Subsystem2/1(DQ)
  abc-dq1/1(DQ) -> Voltage equations/2(vdqr)
  Subsystem2/1(ABC) -> ir_KLM/1
  Constant1/1 -> Subsystem2/2(theta)
  Subsystem1/1(ABC) -> is_UVW/1
  Constant/1 -> abc-dq1/2(theta)
  vr_KLM/1 -> abc-dq1/1(ABC)
  Gain1/1 -> Voltage equations/3(omega)
  omg_mec/1 -> Gain1/1
  [theta] -> Subsystem1/2(theta)
  Voltage equations/1(idqs) -> Subsystem1/1(DQ)
  abc-dq/1(DQ) -> Voltage equations/1(vdqs)
  vs_UVW/1 -> abc-dq/1(ABC)
  [theta] -> abc-dq/2(theta)

== system wt_blockset_beta/Electrical Machinery/Simulink Blocks  based Models/Wound Rotor Induction Machine with Deep Bar Effect  ==
  vs_UVW : Inport
  vr_KLM : Inport  Port=2
  omg_mec : Inport  Port=3
  Constant : Constant  Value=0
  Constant1 : Constant  Value=0
  Gain1 : Gain  Gain=p  SaturateOnIntegerOverflow=on
  Subsystem1 : Subsystem
  Subsystem2 : Subsystem
  Voltage equations : Subsystem
  abc-dq : Subsystem
  abc-dq1 : Subsystem
  is_UVW : Outport  InitialOutput=0
  ir_KLM : Outport  Port=2  InitialOutput=0
  Te : Outport  Port=3  InitialOutput=0
  wires:
  Voltage equations/3(Te) -> Te/1
  Voltage equations/2(idqr) -> Subsystem2/1(DQ)
  abc-dq1/1(DQ) -> Voltage equations/2(vdqr)
  Subsystem2/1(ABC) -> ir_KLM/1
  Constant1/1 -> Subsystem2/2(theta)
  Subsystem1/1(ABC) -> is_UVW/1
  Constant/1 -> abc-dq1/2(theta)
  vr_KLM/1 -> abc-dq1/1(ABC)
  Gain1/1 -> Voltage equations/3(omega)
  omg_mec/1 -> Gain1/1
  [theta] -> Subsystem1/2(theta)
  Voltage equations/1(idqs) -> Subsystem1/1(DQ)
  abc-dq/1(DQ) -> Voltage equations/1(vdqs)
  vs_UVW/1 -> abc-dq/1(ABC)
  [theta] -> abc-dq/2(theta)

== system wt_blockset_beta/Measurements/Phase Locked Loop/PI anti wind-up2 ==
  ref : Inport
  1/T : Gain  Gain=1/Ti  SaturateOnIntegerOverflow=on
  Integrator : Integrator  InitialCondition=init_cond
  P1 : Gain  Gain=K  SaturateOnIntegerOverflow=on
  P2 : Gain  Orientation=left  Gain=ka  SaturateOnIntegerOverflow=on
  Saturation : Saturate  UpperLimit=maxim  LowerLimit=-maxim
  Sum1 : Sum  Inputs=|+-  SaturateOnIntegerOverflow=on  InputSameDT=on
  Sum2 : Sum  Inputs=++|  SaturateOnIntegerOverflow=on  InputSameDT=on
  Sum4 : Sum  Orientation=left  Inputs=+-|  SaturateOnIntegerOverflow=on  InputSameDT=on
  out : Outport  InitialOutput=0
  wires:
  Saturation/1 -> Sum4/2, out/1
  Sum4/1 -> P2/1
  Sum2/1 -> Saturation/1, Sum4/1
  P1/1 -> Sum2/1, Sum1/1
  ref/1 -> P1/1
  1/T/1 -> Integrator/1
  Integrator/1 -> Sum2/2
  Sum1/1 -> 1/T/1
  P2/1 -> Sum1/2

== system wt_blockset_beta/Measurements/power spectra/Spectrum Scope ==
  In1 : Inport
  Data Type Conversion : DataTypeConversion  DataType=double  SaturateOnIntegerOverflow=on
  Frame Scope : S-Function  FunctionName=sdspfscope2  Parameters=s
  Frame Status Conversion : dspsigattribs/Frame Status Conversion  growRefPort=off  outframe=Sample-based
  Optional Buffering : Subsystem  mask(Replaceable Contents){oname=Buffer, osrc=dspbuff3/Buffer, oargs={'N','BufferSize','V','Overlap','ic','0'}, replace=strcmp(UseBuffer,'off')}
      mask prompts: oname "Relative name of blocks to replace:"; osrc "Simulink path to each source block:"; oargs "Parameter/value pairs to each block:"; replace "Replace with short-circuit:"
      mask help: Configurable subsystem holding blocks which may be replaced by virtual short-circuits (muxes) when not needed.
      mask init:
      | opts.name = oname; opts.src = osrc; opts.args = oargs;
      | dspskipblk(gcb,opts,replace);
  Short-Time FFT : dspspect3/Short-Time FFT  wintype=Hann  Rs=50  beta=5  winsamp=Periodic  inheritFFT=off  fftsize=FFTlength  navg=numAvg
  wires:
  Frame Status Conversion/1 -> Frame Scope/1
  Short-Time FFT/1 -> Frame Status Conversion/1
  In1/1 -> Optional Buffering/1(In)
  Optional Buffering/1(Out) -> Data Type Conversion/1
  Data Type Conversion/1 -> Short-Time FFT/1

== system wt_blockset_beta/Mechanical Components/Wind Model SB-1/Kaimal_Filter_1 ==
  in_1 : Inport
  Gain : Gain  Gain=trans/sqrt(2)  SaturateOnIntegerOverflow=on
  Transfer Fcn : TransferFcn  Numerator=[0.0182*c^2 1.3653*c 0.9846]  Denominator=[1.3463*c^2 3.7593*c 1]
  Unit Delay : UnitDelay  SampleTime=T_sample
  out_1 : Outport
  wires:
  Unit Delay/1 -> Transfer Fcn/1
  Gain/1 -> out_1/1
  in_1/1 -> Unit Delay/1
  Transfer Fcn/1 -> Gain/1

== system wt_blockset_beta/Mechanical Components/Wind Model SB-1/Kaimal_Filter_2 ==
  in_1 : Inport
  Gain : Gain  Gain=trans/sqrt(2)  SaturateOnIntegerOverflow=on
  Transfer Function : TransferFcn  Numerator=[0.0182*c^2 1.3653*c 0.9846]  Denominator=[1.3463*c^2 3.7593*c 1]
  Unit Delay : UnitDelay  SampleTime=T_sample
  out_1 : Outport
  wires:
  Unit Delay/1 -> Transfer Function/1
  Gain/1 -> out_1/1
  in_1/1 -> Unit Delay/1
  Transfer Function/1 -> Gain/1

== system wt_blockset_beta/Mechanical Components/Wind Model SB-1/Kaimal_Filter_3 ==
  in_1 : Inport
  Gain : Gain  Gain=trans/sqrt(2)  SaturateOnIntegerOverflow=on
  Transfer Fcn : TransferFcn  Numerator=[0.0182*c^2 1.3653*c 0.9846]  Denominator=[1.3463*c^2 3.7593*c 1]
  Unit Delay : UnitDelay  SampleTime=T_sample
  out_1 : Outport
  wires:
  Unit Delay/1 -> Transfer Fcn/1
  Gain/1 -> out_1/1
  in_1/1 -> Unit Delay/1
  Transfer Fcn/1 -> Gain/1

== system wt_blockset_beta/Mechanical Components/Wind Model SB-1/White Noise_1 ==
  Gain : Gain  Gain=[sqrt(Cov)]/[sqrt(Ts)]  SaturateOnIntegerOverflow=on
  White Noise : RandomNumber  Seed=seed  SampleTime=Ts
  Zero-Order Hold : ZeroOrderHold  SampleTime=Ts
  Out_1 : Outport
  wires:
  White Noise/1 -> Zero-Order Hold/1
  Gain/1 -> Out_1/1
  Zero-Order Hold/1 -> Gain/1

== system wt_blockset_beta/Mechanical Components/Wind Model SB-1/White Noise_2 ==
  Gain : Gain  Gain=[sqrt(Cov)]/[sqrt(Ts)]  SaturateOnIntegerOverflow=on
  White Noise : RandomNumber  Seed=seed  SampleTime=Ts
  Zero-Order Hold : ZeroOrderHold  SampleTime=Ts
  Out_1 : Outport
  wires:
  White Noise/1 -> Zero-Order Hold/1
  Gain/1 -> Out_1/1
  Zero-Order Hold/1 -> Gain/1

== system wt_blockset_beta/Mechanical Components/Wind Model SB-1/White Noise_3 ==
  Gain : Gain  Gain=[sqrt(Cov)]/[sqrt(Ts)]  SaturateOnIntegerOverflow=on
  White Noise : RandomNumber  Seed=seed  SampleTime=Ts
  Zero-Order Hold : ZeroOrderHold  SampleTime=Ts
  Out_1 : Outport
  wires:
  White Noise/1 -> Zero-Order Hold/1
  Gain/1 -> Out_1/1
  Zero-Order Hold/1 -> Gain/1

== system wt_blockset_beta/Mechanical Components/Wind Model SB-2/3rd_Harmonic_Filter1 ==
  avg_wind : Inport
  in_1 : Inport  Port=2
  3rd harmonic Filter : Subsystem
  Unit Delay : UnitDelay  SampleTime=T_sample
  out_1 : Outport
  wires:
  Unit Delay/1 -> 3rd harmonic Filter/2(In)
  in_1/1 -> Unit Delay/1
  avg_wind/1 -> 3rd harmonic Filter/1(avg_wind)
  3rd harmonic Filter/1(Out) -> out_1/1
